simulink model "test_smlk"  (R2023a)
settings: Solver=FixedStepAuto  StartTime=0.0  StopTime=inf  RelTol=1e-3
undefined symbols (not defined in the file or in its folder): angular, linear
libraries: ros2lib x13, robotcorelib x3, robotgazebolib x1
settings Model: Creator=johvany  LastModifiedBy=l15
settings OptimizationCC: EnhancedBackFolding=on  PassReuseOutputArgsAs=Individual arguments  ZeroExternalMemoryAtStartup=off  ZeroInternalMemoryAtStartup=off  MaxStackSize=64  OptimizeBlockOrder=speed  DifferentSizesBufferReuse=on  OptimizationCustomize=off  EfficientTunableParamExpr=on
settings DebuggingCC: ParameterTunabilityLossMsg=error
settings HardwareCC: ProdBitPerLong=64  ProdHWDeviceType=Intel->x86-64 (Linux 64)  UseEmbeddedCoderFeatures=off
settings SFSimCC: MATLABDynamicMemAlloc=off
settings RTWCC: Description=Embedded Coder  SystemTargetFile=ert.tlc  HardwareBoard=Robot Operating System 2 (ROS 2)  TLCOptions="-aInlineSetEventsForThisBaseRateFcn=TLC_FALSE -aSuppressMultiTaskScheduler=TLC_FALSE  -aRateBasedStepFcn=0"  TemplateMakefile=ert_default_tmf  Toolchain=Colcon Tools  TargetLang=C++
settings CodeAppCC: ForceParamTrailComments=on  IgnoreCustomStorageClasses=off  OperatorAnnotations=on  SimulinkDataObjDesc=on  SFDataObjDesc=on  InsertBlockDesc=on
settings ERTTargetCC: CodeInterfacePackaging=C++ class  SupportNonInlinedSFcns=on  RootIOFormat=Structure reference

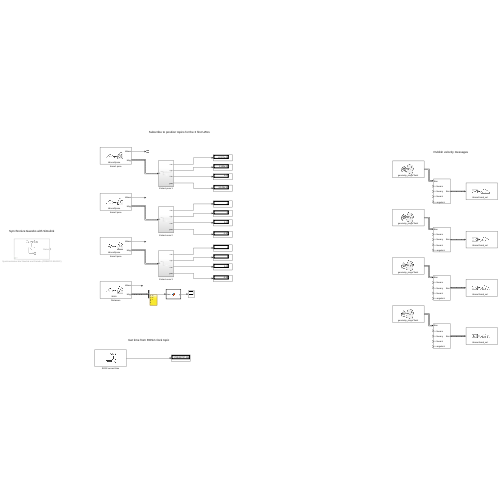
[thumbnail: Simulink's stored preview of the top-level diagram]
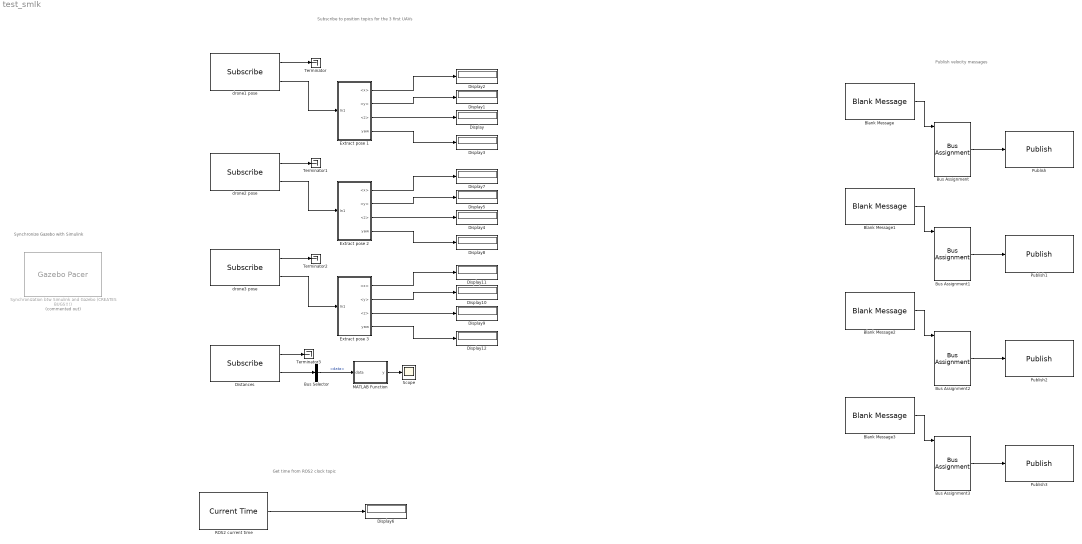
== system test_smlk ==
  note: Publish velocity messages
  note: Subscribe to position topics for the 3 first UAVs
  note: Get time from ROS2 clock topic
  note: Synchronize Gazebo with Simulink
  Blank Message{,1..3} (4 alike) : ros2lib/Blank Message  messageClass=Message  entityType=geometry_msgs/Twist  messageType=geometry_msgs/Twist  SampleTime=inf
  Bus Assignment{,1..3} (4 alike) : BusAssignment  AssignedSignals=linear.x,linear.y,linear.z,angular.z
  Bus Selector : BusSelector  OutputSignals=data
  Display{,1..12} (13 alike) : Display
  Distances : ros2lib/Subscribe  topicSource=Select from ROS network  topic=/dists  messageType=std_msgs/Float32MultiArray  sampleTime=-1  QOSHistory=Keep last  QOSDepth=1  QOSReliability=Reliable  QOSDurability=Volatile
  Extract pose 1 : Subsystem
  Extract pose 2 : Subsystem
  Extract pose 3 : Subsystem
  MATLAB Function : MATLAB Function  TreatAsAtomicUnit=on
  Publish : ros2lib/Publish  topicSource=Select from ROS network  topic=/drone1/cmd_vel  messageType=geometry_msgs/Twist  QOSHistory=Keep last  QOSDepth=1  QOSReliability=Reliable  QOSDurability=Volatile
  Publish1 : ros2lib/Publish  topicSource=Select from ROS network  topic=/drone2/cmd_vel  messageType=geometry_msgs/Twist  QOSHistory=Keep last  QOSDepth=1  QOSReliability=Reliable  QOSDurability=Volatile
  Publish2 : ros2lib/Publish  topicSource=Select from ROS network  topic=/drone3/cmd_vel  messageType=geometry_msgs/Twist  QOSHistory=Keep last  QOSDepth=1  QOSReliability=Reliable  QOSDurability=Volatile
  Publish3 : ros2lib/Publish  topicSource=Select from ROS network  topic=/drone4/cmd_vel  messageType=geometry_msgs/Twist  QOSHistory=Keep last  QOSDepth=1  QOSReliability=Reliable  QOSDurability=Volatile
  ROS2 current time : ros2lib/Current Time  OutputFormat=double  SampleTime=-1  ModelName=test_smlk
  Scope : Scope
  Synchronization btw Simulink and Gazebo (CREATES BUGS!!!) : robotgazebolib/Gazebo Pacer  Commented=on  ResetBehavior=Reset Gazebo simulation time  SampleTime=0.001
  Terminator{,1..3} (4 alike) : Terminator
  drone1 pose : ros2lib/Subscribe  topicSource=Select from ROS network  topic=/drone1/pose  messageType=geometry_msgs/PoseStamped  sampleTime=-1  QOSHistory=Keep last  QOSDepth=1  QOSReliability=Reliable  QOSDurability=Volatile
  drone2 pose : ros2lib/Subscribe  topicSource=Select from ROS network  topic=/drone2/pose  messageType=geometry_msgs/PoseStamped  sampleTime=-1  QOSHistory=Keep last  QOSDepth=1  QOSReliability=Reliable  QOSDurability=Volatile
  drone3 pose : ros2lib/Subscribe  topicSource=Select from ROS network  topic=/drone3/pose  messageType=geometry_msgs/PoseStamped  sampleTime=-1  QOSHistory=Keep last  QOSDepth=1  QOSReliability=Reliable  QOSDurability=Volatile
  wires:
  drone1 pose/1 -> Terminator/1
  ROS2 current time/1 -> Display6/1
  drone1 pose/2 -> Extract pose 1/1(In1)
  Extract pose 1/1(<x>) -> Display2/1
  Extract pose 1/2(<y>) -> Display1/1
  Extract pose 1/3(<z>) -> Display/1
  Extract pose 1/4(yaw) -> Display3/1
  Extract pose 2/3(<z>) -> Display4/1
  drone2 pose/2 -> Extract pose 2/1(In1)
  Extract pose 2/1(<x>) -> Display7/1
  Extract pose 2/4(yaw) -> Display8/1
  Extract pose 2/2(<y>) -> Display5/1
  drone2 pose/1 -> Terminator1/1
  Extract pose 3/3(<z>) -> Display9/1
  drone3 pose/2 -> Extract pose 3/1(In1)
  Extract pose 3/1(<x>) -> Display11/1
  Extract pose 3/4(yaw) -> Display12/1
  Extract pose 3/2(<y>) -> Display10/1
  drone3 pose/1 -> Terminator2/1
  Blank Message/1 -> Bus Assignment/1
  Bus Assignment/1 -> Publish/1
  Blank Message1/1 -> Bus Assignment1/1
  Bus Assignment1/1 -> Publish1/1
  Blank Message2/1 -> Bus Assignment2/1
  Bus Assignment2/1 -> Publish2/1
  Blank Message3/1 -> Bus Assignment3/1
  Bus Assignment3/1 -> Publish3/1
  Distances/1 -> Terminator3/1
  Distances/2 -> Bus Selector/1
  Bus Selector/1 -> MATLAB Function/1(data)  "<data>"
  MATLAB Function/1(y) -> Scope/1

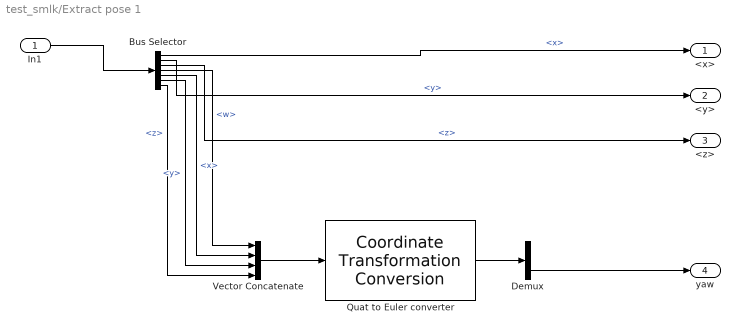
== system test_smlk/Extract pose 1 ==
  In1 : Inport
  Bus Selector : BusSelector  OutputSignals=pose.position.x,pose.position.y,pose.position.z,pose.orientation.w,pose.orientation.x,pose.orientation.y,pose.orientation.z
  Demux : Demux  Outputs=3
  Quat to Euler converter : robotcorelib/Coordinate Transformation Conversion  InputRepresentation=Quaternion  InputEulerSequence=ZYX  ShowTrVecInputPort=on  OutputRepresentation=Euler Angles  OutputEulerSequence=XYZ  ShowTrVecOutputPort=on  SimulateUsing=Interpreted execution
      settings: LibrarySourceBlock=roslib/Utilities/Coordinate Transformation Conversion
  Vector Concatenate : Concatenate  NumInputs=4
  <x> : Outport
  <y> : Outport  Port=2
  <z> : Outport  Port=3
  yaw : Outport  Port=4
  wires:
  Bus Selector/5 -> Vector Concatenate/2  "<x>"
  Quat to Euler converter/1 -> Demux/1
  Demux/3 -> yaw/1
  Bus Selector/6 -> Vector Concatenate/3  "<y>"
  Bus Selector/1 -> <x>/1  "<x>"
  Bus Selector/7 -> Vector Concatenate/4  "<z>"
  Vector Concatenate/1 -> Quat to Euler converter/1
  In1/1 -> Bus Selector/1
  Bus Selector/4 -> Vector Concatenate/1  "<w>"
  Bus Selector/2 -> <y>/1  "<y>"
  Bus Selector/3 -> <z>/1  "<z>"

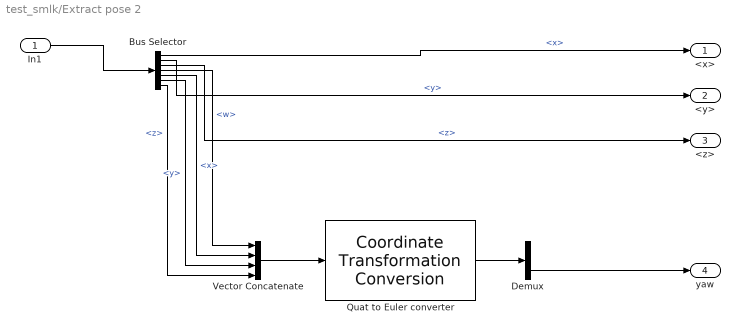
== system test_smlk/Extract pose 2 ==
  In1 : Inport
  Bus Selector : BusSelector  OutputSignals=pose.position.x,pose.position.y,pose.position.z,pose.orientation.w,pose.orientation.x,pose.orientation.y,pose.orientation.z
  Demux : Demux  Outputs=3
  Quat to Euler converter : robotcorelib/Coordinate Transformation Conversion  InputRepresentation=Quaternion  InputEulerSequence=ZYX  ShowTrVecInputPort=on  OutputRepresentation=Euler Angles  OutputEulerSequence=XYZ  ShowTrVecOutputPort=on  SimulateUsing=Interpreted execution
      settings: LibrarySourceBlock=roslib/Utilities/Coordinate Transformation Conversion
  Vector Concatenate : Concatenate  NumInputs=4
  <x> : Outport
  <y> : Outport  Port=2
  <z> : Outport  Port=3
  yaw : Outport  Port=4
  wires:
  Bus Selector/5 -> Vector Concatenate/2  "<x>"
  Quat to Euler converter/1 -> Demux/1
  Demux/3 -> yaw/1
  Bus Selector/6 -> Vector Concatenate/3  "<y>"
  Bus Selector/1 -> <x>/1  "<x>"
  Bus Selector/7 -> Vector Concatenate/4  "<z>"
  Vector Concatenate/1 -> Quat to Euler converter/1
  In1/1 -> Bus Selector/1
  Bus Selector/4 -> Vector Concatenate/1  "<w>"
  Bus Selector/2 -> <y>/1  "<y>"
  Bus Selector/3 -> <z>/1  "<z>"

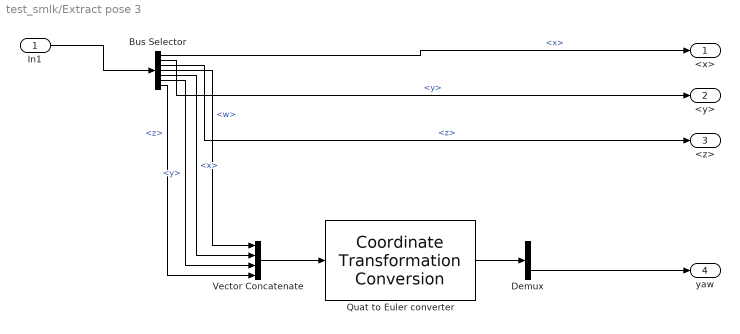
== system test_smlk/Extract pose 3 ==
  In1 : Inport
  Bus Selector : BusSelector  OutputSignals=pose.position.x,pose.position.y,pose.position.z,pose.orientation.w,pose.orientation.x,pose.orientation.y,pose.orientation.z
  Demux : Demux  Outputs=3
  Quat to Euler converter : robotcorelib/Coordinate Transformation Conversion  InputRepresentation=Quaternion  InputEulerSequence=ZYX  ShowTrVecInputPort=on  OutputRepresentation=Euler Angles  OutputEulerSequence=XYZ  ShowTrVecOutputPort=on  SimulateUsing=Interpreted execution
      settings: LibrarySourceBlock=roslib/Utilities/Coordinate Transformation Conversion
  Vector Concatenate : Concatenate  NumInputs=4
  <x> : Outport
  <y> : Outport  Port=2
  <z> : Outport  Port=3
  yaw : Outport  Port=4
  wires:
  Bus Selector/5 -> Vector Concatenate/2  "<x>"
  Quat to Euler converter/1 -> Demux/1
  Demux/3 -> yaw/1
  Bus Selector/6 -> Vector Concatenate/3  "<y>"
  Bus Selector/1 -> <x>/1  "<x>"
  Bus Selector/7 -> Vector Concatenate/4  "<z>"
  Vector Concatenate/1 -> Quat to Euler converter/1
  In1/1 -> Bus Selector/1
  Bus Selector/4 -> Vector Concatenate/1  "<w>"
  Bus Selector/2 -> <y>/1  "<y>"
  Bus Selector/3 -> <z>/1  "<z>"

== matlab function test_smlk/MATLAB Function ==
  data: data input; y output
function y = fcn(data)

DATA = data(1:20);
d1 = DATA(1);
d2 = DATA(2);
d3 = DATA(3);
y = [d1;d2;d3];
